simulink library "simeventstranslate1"  (Simulink 7.2)
settings: Solver=ode45  SolverMode=SingleTasking  StartTime=0.0  StopTime=10.0  RelTol=1e-3
undefined symbols (not defined in the file or in its folder): des_support, gcbh
libraries: des_sfun_lib x3
settings Model: Creator=mclune  LastModifiedBy=Liw  ExtModeAutoUpdateStatusClock=off

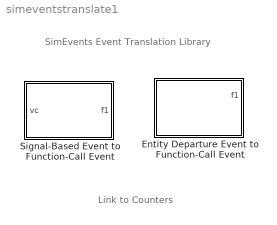
== system simeventstranslate1 ==
  note: SimEvents Event Translation Library
  note: Link to Counters
  Entity Departure Event to Function-Call Event : Subsystem  Priority=1  LoadFcn=des_support('desLoadFcn',gcbh)  StartFcn=des_support('desStartFcn',gcbh)  StopFcn=des_support('desStopFcn',gcbh)  mask(Entity Departure Event to Function-Call Event){TimingFunctionCallF1=After entity departure, EnableE1Port=off, EnableF2Port=off, TimingFunctionCallF2=Before entity departure, EnableE2Port=off, StatNumberDeparted=Off, StatNumberF1Calls=Off, StatNumberF2Calls=Off, IsInsideAFB=off}
      mask prompts: TimingFunctionCallF1 "Timing of function call f1:"; EnableE1Port "Suppress function call f1 if enable signal e1 is not positive"; EnableF2Port "Generate optional function call f2 after function call f1"; TimingFunctionCallF2 "Timing of function call f2:"; EnableE2Port "Suppress function call f2 if enable signal e2  is not positive"; StatNumberDeparted "Number of entities departed, #d:"; StatNumberF1Calls "Number of f1 function calls, #f1:"; StatNumberF2Calls "Number of f2 function calls, #f2:"; IsInsideAFB "The block is inside a Attribute Function Block"
      mask help: Convert an entity departure event into one or two function calls. The block can suppress a function call based on the corresponding enable signal.
      mask init:
      | des_entityfcncallmask(gcb, 'init','apply')
      settings: CopyFcn=des_support('desCopyFcn',gcbh)  DeleteFcn=des_support('desDeleteFcn',gcbh)  UndoDeleteFcn=des_support('desUndoDeleteFcn',gcbh)  ModelCloseFcn=des_support('desModelCloseFcn',gcbh)  PreSaveFcn=des_support('desPreSaveFcn',gcbh)  PostSaveFcn=des_support('desPostSaveFcn',gcbh)  NameChangeFcn=des_support('desNameChangeFcn',gcbh)  CloseFcn=des_support('desCloseFcn',gcbh)  ErrorFcn=des_error_redirect
      mask Help: helpview(simeventsbhelp)
      mask StyleString: popup(Before entity departure|After entity departure),checkbox,checkbox,popup(Before entity departure|After entity departure),checkbox,popup(Off|On|Upon stop or pause),popup(Off|On|Upon stop or pause),popup(Off|On|Upon stop or pause),checkbox
      mask CallbackString: des_entityfcncallmask(gcb,'cbFcnCallUpon','noapply');|des_entityfcncallmask(gcb,'cbEnableE1Port','noapply');|des_entityfcncallmask(gcb,'cbEnableF2Port','noapply');||des_entityfcncallmask(gcb,'cbEnableE2Port','noapply');|des_entityfcncallmask(gcb,'cbStatNumberDeparted','noapply');|des_entityfcncallmask(gcb,'cbStatNumberF1Calls','noapply');|des_entityfcncallmask(gcb,'cbStatNumberF2Calls','noapply');|
      mask TabNameString: Function Call,Function Call,Function Call,Function Call,Function Call,Statistics,Statistics,Statistics,Statistics
      mask Display:
      | image(des_iconLoad('transEntToFunc.jpg'),'center');
      | port_label('LConn',1,'IN');
      | port_label('RConn',1,'OUT');
      | port_label('output',1,'f1');
  Signal-Based Event to Function-Call Event : Subsystem  Priority=1  LoadFcn=des_support('desLoadFcn',gcbh)  StartFcn=des_support('desStartFcn',gcbh)  StopFcn=des_support('desStopFcn',gcbh)  mask(Signal-Based Event to Function-Call Event){GenerateFunctionCallUpon=Change in signal from port vc, SignalEdgeOption=Rising, EnableE1Port=off, EnableF2Port=off, EnableE2Port=off, SpecifyEventPriority=off, PriorityFunctionCall=200, FunctionCallDelayFrom=Dialog, DelayFunctionCall=0, StatNumberF1Calls=Off, StatNumberF2Calls=Off, MaskBlockType=none}
      mask prompts: GenerateFunctionCallUpon "Generate function call only upon:"; SignalEdgeOption "Type of change in signal value:"; EnableE1Port "Suppress function call f1 if enable signal e1 is not positive"; EnableF2Port "Generate optional f2 function call"; EnableE2Port "Suppress function call f2 if enable signal e2  is not positive"; SpecifyEventPriority "Resolve simultaneous signal updates according to event priority"; PriorityFunctionCall "Event priority:"; FunctionCallDelayFrom "Function-call delay from:"; DelayFunctionCall "Function-call time delay:"; StatNumberF1Calls "Number of f1 function calls, #f1:"; StatNumberF2Calls "Number of f2 function calls, #f2:"; MaskBlockType "Masked block type:"
      mask help:
      | Translate a signal-based event or an input function call into one or two output function calls. Use dialog parameters to specify the type of event the block converts and whether the block suppresses its output under certain conditions.
      |
      | If the block issues function calls at both the f1 and optional f2 output ports, then it issues the f1 call first.
      mask init:
      | des_fcncallmask(gcb, 'init','apply')
      settings: CopyFcn=des_support('desCopyFcn',gcbh)  DeleteFcn=des_support('desDeleteFcn',gcbh)  UndoDeleteFcn=des_support('desUndoDeleteFcn',gcbh)  ModelCloseFcn=des_support('desModelCloseFcn',gcbh)  PreSaveFcn=des_support('desPreSaveFcn',gcbh)  PostSaveFcn=des_support('desPostSaveFcn',gcbh)  NameChangeFcn=des_support('desNameChangeFcn',gcbh)  CloseFcn=des_support('desCloseFcn',gcbh)  ErrorFcn=des_error_redirect
      mask Help: helpview(simeventsbhelp)
      mask StyleString: popup(Sample time hit from port ts|Trigger from port tr|Change in signal from port vc|Function call from port fcn),popup(Rising|Falling|Either),checkbox,checkbox,checkbox,checkbox,edit,popup(Dialog|Signal port t),edit,popup(Off|On|Upon stop or pause),popup(Off|On|Upon stop or pause),popup(none|DESS_EVENT_PORT|DESS_DATA_PORT|TOWKSPC_HAS_IC|TOWKSPC_NO_IC)
      mask CallbackString: des_fcncallmask(gcb,'cbFcnCallUpon','noapply');||des_fcncallmask(gcb,'cbEnableE1Port','noapply');|des_fcncallmask(gcb,'cbEnableF2Port','noapply');|des_fcncallmask(gcb,'cbEnableE2Port','noapply');|des_fcncallmask(gcb,'cbSpecifyEventPriority','noapply');||des_fcncallmask(gcb,'cbFcnCallDelayFrom','noapply');||des_fcncallmask(gcb,'cbStatNumberF1Calls','noapply');|des_fcncallmask(gcb,'cbStatNumberF2Calls','noapply');|
      mask TabNameString: Function Call,Function Call,Function Call,Function Call,Function Call,Timing,Timing,Timing,Timing,Statistics,Statistics,Statistics
      mask Display:
      | image(des_iconLoad('transSigToFunc.jpg'),'center');
      | port_label('input',1,'vc');
      | port_label('output',1,'f1');

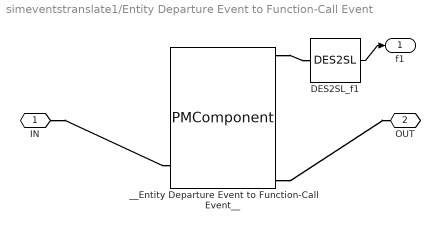
== system simeventstranslate1/Entity Departure Event to Function-Call Event ==
  DES2SL_f1 : des_sfun_lib/DES2SL  SystemSampleTime=-1  PortType=desPortIn  PhysicalDomain=simevents  SubClassName=DES_DES2SL  timingControl=FunctionCall  execIndex=0  multipleOutputs=off  updateBeforeRead=off  InitValue=0  sampleTime=-1  offsetTime=0  idxBlockMR=0  IsMonitorOnly=off  dimsInfo=1
  __Entity Departure Event to Function-Call Event__ : PMComponent  PhysicalDomain=simevents  SubClassName=DES_ENTITYFUNCTIONCALL  LeftPortType=desPortIn  RightPortType=desPortOut  LConnTagsString=DI|DI|DI  RConnTagsString=DO|DO|DO|DO|DO|DO
      mask Display:
      | port_label('LConn',1,'e1');
      | port_label('LConn',2,'e2');
      | port_label('LConn',3,'IN');
      | port_label('RConn',1,'f1');
      | port_label('RConn',2,'f2');
      | port_label('RConn',3,'#d');
      | port_label('RConn',4,'#f1');
      | port_label('RConn',5,'#f2');
      | port_label('RConn',6,'OUT');
  IN : PMIOPort  Port=1  Side=Left
  OUT : PMIOPort  Orientation=left  Port=2  Side=Right
  f1 : Outport  OutDataType=sfix(16)  OutScaling=2^0
  wires:
  DES2SL_f1/1 -> f1/1
  connections:
  IN/RConn1 -- __Entity Departure Event to Function-Call Event__/LConn3
  __Entity Departure Event to Function-Call Event__/RConn6 -- OUT/RConn1
  __Entity Departure Event to Function-Call Event__/RConn1 -- DES2SL_f1/LConn1

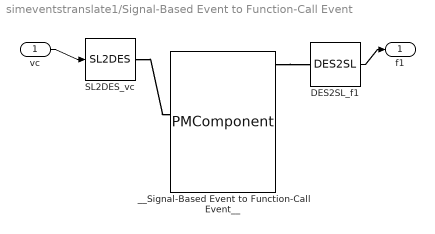
== system simeventstranslate1/Signal-Based Event to Function-Call Event ==
  vc : Inport  PortDimensions=1  DataType=double  OutDataType=sfix(16)  OutScaling=2^0  OutDataTypeStr=double
  DES2SL_f1 : des_sfun_lib/DES2SL  SystemSampleTime=-1  PortType=desPortIn  PhysicalDomain=simevents  SubClassName=DES_DES2SL  timingControl=FunctionCall  execIndex=0  multipleOutputs=off  updateBeforeRead=off  InitValue=0  sampleTime=-1  offsetTime=0  idxBlockMR=0  IsMonitorOnly=off  dimsInfo=1
  SL2DES_vc : des_sfun_lib/SL2DES  SystemSampleTime=-1  PortType=desPortOut  PhysicalDomain=simevents  SubClassName=DES_SL2DES  timingControl=Simulink  execIndex=200  trigger=None  filter=0  updateBeforeRead=off  InitValue=0  initToFactVal=off  sampleTime=-1  offsetTime=0  idxBlockMR=0  IsMonitorOnly=off  dimsInfo=1
  __Signal-Based Event to Function-Call Event__ : PMComponent  PhysicalDomain=simevents  SubClassName=DES_FUNCTIONCALL  LeftPortType=desPortIn  RightPortType=desPortOut  LConnTagsString=DI|DI|DI|DI|DI|DI|DI|DI  RConnTagsString=DO|DO|DO|DO|DO
      mask Display:
      | port_label('LConn',1,'t');
      | port_label('LConn',2,'ts');
      | port_label('LConn',3,'tr');
      | port_label('LConn',4,'vc');
      | port_label('LConn',5,'fcn');
      | port_label('LConn',6,'e1');
      | port_label('LConn',7,'e2');
      | port_label('LConn',8,'IN');
      | port_label('RConn',1,'f1');
      | port_label('RConn',2,'f2');
      | port_label('RConn',3,'#f1');
      | port_label('RConn',4,'#f2');
      | port_label('RConn',5,'OUT');
  f1 : Outport  OutDataType=sfix(16)  OutScaling=2^0
  wires:
  DES2SL_f1/1 -> f1/1
  vc/1 -> SL2DES_vc/1
  connections:
  __Signal-Based Event to Function-Call Event__/RConn1 -- DES2SL_f1/LConn1
  SL2DES_vc/RConn1 -- __Signal-Based Event to Function-Call Event__/LConn4
